simulink model "Clamper"  (R2018a)
settings: Solver=VariableStepAuto  StartTime=0.0  StopTime=0.5  RelTol=1e-3
libraries: powerlib x28, simulink x2
settings Model: Creator=Sadat Zubin Shah  LastModifiedBy=Sadat Zubin Shah

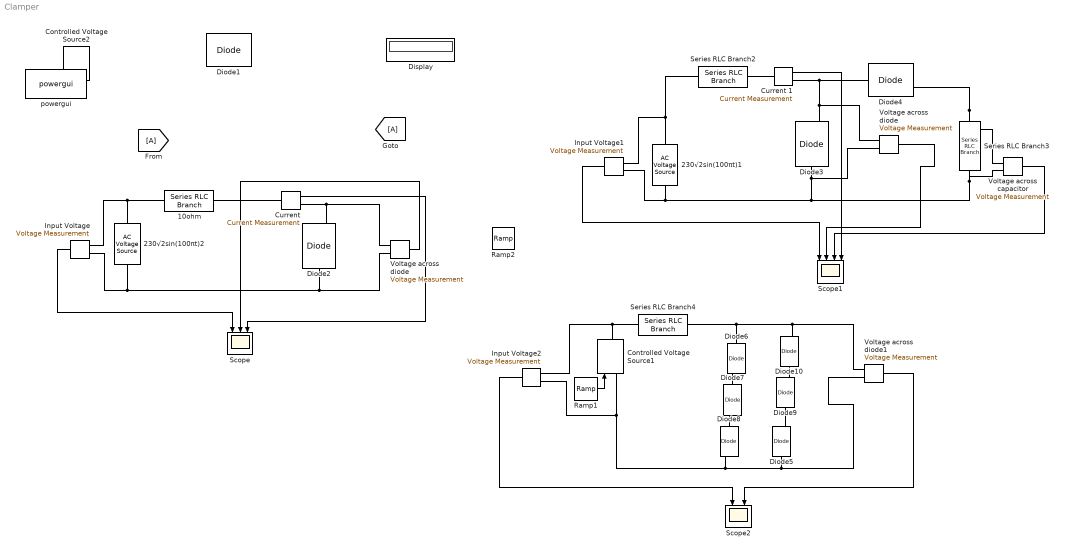
== system Clamper ==
  10ohm : powerlib/Elements/Series RLC Branch  LConnTagsString=__new0  RConnTagsString=__new0  BranchType=R  Resistance=10  Inductance=1e-3  SetiL0=off  InitialCurrent=0  Capacitance=1e-6  Setx0=off  InitialVoltage=0  Measurements=None
  230√2sin(100πt)1 : powerlib/Electrical Sources/AC Voltage Source  Amplitude=230*sqrt(2)  Phase=0  Frequency=50  SampleTime=0  Measurements=None  BusType=swing  Pref=10e3  Qref=0  Qmin=-inf  Qmax=+inf
  230√2sin(100πt)2 : powerlib/Electrical Sources/AC Voltage Source  Amplitude=230*sqrt(2)  Phase=0  Frequency=50  SampleTime=0  Measurements=None  BusType=swing  Pref=10e3  Qref=0  Qmin=-inf  Qmax=+inf
  Controlled Voltage Source1 : powerlib/Electrical Sources/Controlled Voltage Source  Initialize=off  Source_Type=AC  Amplitude=0  Phase=0  Frequency=0  Measurements=None
  Controlled Voltage Source2 : powerlib/Electrical Sources/Controlled Voltage Source  Initialize=off  Source_Type=AC  Amplitude=0  Phase=0  Frequency=0  Measurements=None
  "Current " : powerlib/Measurements/Current Measurement  PhasorSimulation=off  OutputType=Complex  PSBequivalent=0
  Current 1 : powerlib/Measurements/Current Measurement  PhasorSimulation=off  OutputType=Complex  PSBequivalent=0
  Diode{1..10} (10 alike) : powerlib/Power Electronics/Diode  Ron=0.001  Lon=0  Vf=0.7  IC=0  UseSnubber=0  Rs=500  Cs=250e-9  Measurements=on
  Display : Display
  Input Voltage : powerlib/Measurements/Voltage Measurement  PhasorSimulation=off  OutputType=Complex  PSBequivalent=0
  Input Voltage1 : powerlib/Measurements/Voltage Measurement  PhasorSimulation=off  OutputType=Complex  PSBequivalent=0
  Input Voltage2 : powerlib/Measurements/Voltage Measurement  PhasorSimulation=off  OutputType=Complex  PSBequivalent=0
  Ramp1 : simulink/Sources/Ramp  slope=10  start=0  InitialOutput=-5  VectorParams1D=off
  Ramp2 : simulink/Sources/Ramp  slope=10  start=0  InitialOutput=0
  Scope : Scope  NumInputPorts=3
  Scope1 : Scope  NumInputPorts=4
  Scope2 : Scope  NumInputPorts=2
  Series RLC Branch2 : powerlib/Elements/Series RLC Branch  LConnTagsString=__new0  RConnTagsString=__new0  BranchType=C  Resistance=10  Inductance=1e-3  SetiL0=off  InitialCurrent=0  Capacitance=1e-3  Setx0=off  InitialVoltage=0  Measurements=None
  Series RLC Branch3 : powerlib/Elements/Series RLC Branch  LConnTagsString=__new0  RConnTagsString=__new0  BranchType=C  Resistance=10  Inductance=1e-3  SetiL0=off  InitialCurrent=0  Capacitance=1e-3  Setx0=off  InitialVoltage=0  Measurements=None
  Series RLC Branch4 : powerlib/Elements/Series RLC Branch  LConnTagsString=__new0  RConnTagsString=__new0  BranchType=R  Resistance=10  Inductance=1e-3  SetiL0=off  InitialCurrent=0  Capacitance=1e-6  Setx0=off  InitialVoltage=0  Measurements=None
  Voltage across capacitor : powerlib/Measurements/Voltage Measurement  PhasorSimulation=off  OutputType=Complex  PSBequivalent=0
  Voltage across diode : powerlib/Measurements/Voltage Measurement  PhasorSimulation=off  OutputType=Complex  PSBequivalent=0
  "Voltage across diode  " : powerlib/Measurements/Voltage Measurement  PhasorSimulation=off  OutputType=Complex  PSBequivalent=0
  Voltage across diode1 : powerlib/Measurements/Voltage Measurement  PhasorSimulation=off  OutputType=Complex  PSBequivalent=0
  powergui : powerlib/powergui  Priority=1  SimulationMode=Discrete  SampleTime=50e-6  frequency=60  Iterations=50  frequencyindice=0  Pbase=100e6  ErrMax=1e-4  UnitsV=kV  UnitsW=MW  buscounter=0  FunctionMessages=off  echomessages=off  EnableUseOfTLC=off  CurrentSourceSwitches=off  DisableSnubberDevices=off  DisableRonSwitches=off  DisableVfSwitches=off  DisplayEquations=off  SolverType=Tustin/Backward Euler (TBE)  Interpol=off  ExternalGateDelay=off  methode=off  Ts=100  x0status=blocks  SPID=on  SwTol=0  HookPort=off  RestoreLinks=warning  ResistiveCurrentMeasurement=off  Frange=[0:2:500]  Ylog=off  Xlog=on  ShowGrid=off  save=off  variable=ZData  structure=0  ZoomFFT=off  StartTime=0.0  cycles=1  DisplayStyle=1  fundamental=60  FreqAxis=off  MaxFrequency=1000  frequencyindicesteady=1  RmsSteady=1  display=off
  wires:
  Input Voltage/1 -> Scope/1
  Voltage across diode/1 -> Scope/2
  "Current "/1 -> Scope/3
  Input Voltage1/1 -> Scope1/1
  "Voltage across diode  "/1 -> Scope1/2
  Voltage across capacitor/1 -> Scope1/3
  Current 1/1 -> Scope1/4
  Voltage across diode1/1 -> Scope2/2
  Input Voltage2/1 -> Scope2/1
  Ramp1/1 -> Controlled Voltage Source1/1
  connections:
  Input Voltage/LConn1 -- 230√2sin(100πt)2/RConn1 -- 10ohm/RConn1
  "Current "/RConn1 -- Voltage across diode/LConn1 -- Diode2/RConn1
  Voltage across diode/LConn2 -- Diode2/LConn1 -- 230√2sin(100πt)2/LConn1 -- Input Voltage/LConn2
  "Current "/LConn1 -- 10ohm/LConn1
  Current 1/RConn1 -- Diode4/LConn1 -- "Voltage across diode  "/LConn1 -- Diode3/RConn1
  Diode4/RConn1 -- Voltage across capacitor/LConn1 -- Series RLC Branch3/RConn1
  230√2sin(100πt)1/LConn1 -- Diode3/LConn1 -- "Voltage across diode  "/LConn2 -- Voltage across capacitor/LConn2 -- Series RLC Branch3/LConn1 -- Input Voltage1/LConn2
  Current 1/LConn1 -- Series RLC Branch2/LConn1
  Input Voltage1/LConn1 -- 230√2sin(100πt)1/RConn1 -- Series RLC Branch2/RConn1
  Input Voltage2/LConn1 -- Series RLC Branch4/RConn1 -- Controlled Voltage Source1/RConn1
  Diode6/LConn1 -- Series RLC Branch4/LConn1 -- Diode10/RConn1 -- Voltage across diode1/LConn1
  Input Voltage2/LConn2 -- Controlled Voltage Source1/LConn1 -- Voltage across diode1/LConn2 -- Diode5/LConn1 -- Diode8/RConn1
  Diode7/LConn1 -- Diode6/RConn1
  Diode8/LConn1 -- Diode7/RConn1
  Diode9/LConn1 -- Diode5/RConn1
  Diode10/LConn1 -- Diode9/RConn1
